simulink model "Lightning_McSeas_Dashboard"  (R2021b)
settings: Solver=VariableStepAuto  StartTime=0.0  StopTime=inf  RelTol=1e-3
undefined symbols (not defined in the file): canChannel
libraries: canlib x10, canmsglib x10
(part 2 of 2)

== system Lightning_McSeas_Dashboard/Battery Definiton ==
  note: Need to add the information for all of the voltages and temperatures maybe
  note: Battery definiton
  CAN Receive : canlib/CAN Receive  BlockHandle=5.0002  Device=MathWorks Virtual 1 (Channel 1)  DeviceMenu=MathWorks Virtual 1 (Channel 1)  ObjConstructor=canChannel('MathWorks', 'Virtual 1', 1)  EnableStandardIDsFilter=off  StdIDsCombo=Allow all  StandardIDs=1536  EnableExtendedIDsFilter=off  ExtIDsCombo=Allow all  ExtendedIDs=0  SampleTime=0.1  MsgsPerTimestep=all  InternalFilterUpdateStatus=on  BusOutput=off
      settings: SourceProductBaseCode=VN
  Dead : Terminator
  GPS Function : Subsystem  TreatAsAtomicUnit=on
  wires:
  CAN Receive/2 -> GPS Function/1(CAN Msg)
  GPS Function/1(Speed) -> Dead/1
  CAN Receive/1 -> GPS Function/Trigger

== system Lightning_McSeas_Dashboard/GPS Definintion ==
  note: GPS definiton
  CAN Receive : canlib/CAN Receive  BlockHandle=72.0009  Device=MathWorks Virtual 1 (Channel 1)  DeviceMenu=MathWorks Virtual 1 (Channel 1)  ObjConstructor=canChannel('MathWorks', 'Virtual 1', 1)  EnableStandardIDsFilter=off  StdIDsCombo=Allow all  StandardIDs=1536  EnableExtendedIDsFilter=off  ExtIDsCombo=Allow all  ExtendedIDs=0  SampleTime=0.1  MsgsPerTimestep=all  InternalFilterUpdateStatus=on  BusOutput=off
      settings: SourceProductBaseCode=VN
  GPS Function : Subsystem  TreatAsAtomicUnit=on
  Speed : Terminator
  wires:
  CAN Receive/2 -> GPS Function/1(CAN Msg)
  GPS Function/1(Speed) -> Speed/1
  CAN Receive/1 -> GPS Function/Trigger

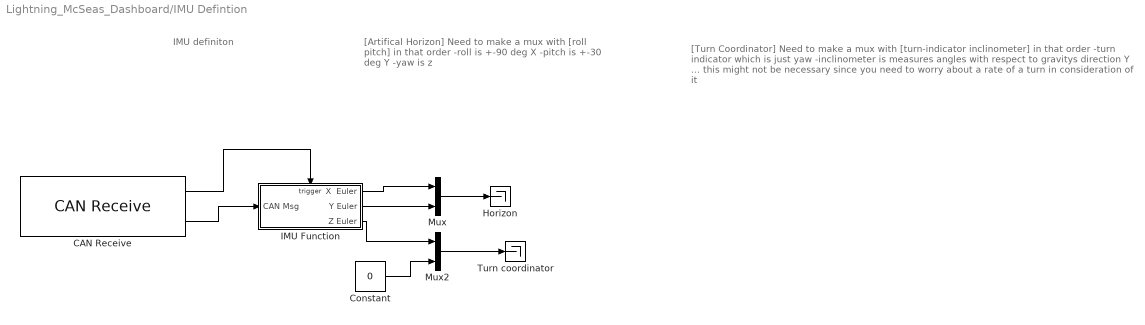
== system Lightning_McSeas_Dashboard/IMU Defintion ==
  note: [Turn Coordinator]
      | Need to make a mux with [turn-indicator inclinometer] in that order
      | -turn indicator which is just yaw
      |
      | -inclinometer is measures angles with respect to gravitys direction Y
      |
      | ... this might not be necessary since you need to worry about a rate of a turn in consideration of it
  note: [Artifical Horizon]
      | Need to make a mux with [roll pitch] in that order
      | -roll is +-90 deg X
      | -pitch is +-30 deg Y
      |
      | -yaw is z
  note: IMU definiton
  CAN Receive : canlib/CAN Receive  BlockHandle=38.0002  Device=MathWorks Virtual 1 (Channel 1)  DeviceMenu=MathWorks Virtual 1 (Channel 1)  ObjConstructor=canChannel('MathWorks', 'Virtual 1', 1)  EnableStandardIDsFilter=off  StdIDsCombo=Allow all  StandardIDs=1536  EnableExtendedIDsFilter=off  ExtIDsCombo=Allow all  ExtendedIDs=0  SampleTime=0.1  MsgsPerTimestep=all  InternalFilterUpdateStatus=on  BusOutput=off
      settings: SourceProductBaseCode=VN
  Constant : Constant  Value=0
  Horizon : Terminator
  IMU Function : Subsystem  TreatAsAtomicUnit=on
  Mux : Mux  Inputs=2
  Mux2 : Mux  Inputs=2
  Turn coordinator : Terminator
  wires:
  CAN Receive/2 -> IMU Function/1(CAN Msg)
  IMU Function/2(Y Euler) -> Mux/2
  IMU Function/3(Z Euler) -> Mux2/1
  CAN Receive/1 -> IMU Function/Trigger
  IMU Function/1(X  Euler) -> Mux/1
  Mux/1 -> Horizon/1
  Mux2/1 -> Turn coordinator/1
  Constant/1 -> Mux2/2

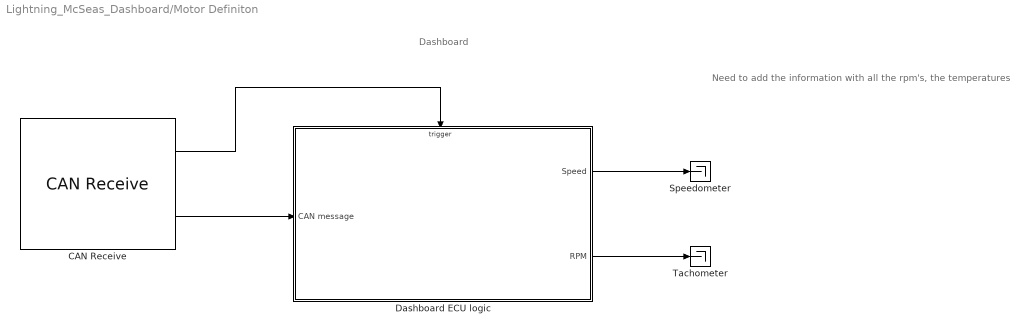
== system Lightning_McSeas_Dashboard/Motor Definiton ==
  note: Need to add the information with all the rpm's, the temperatures
  note: Dashboard
  CAN Receive : canlib/CAN Receive  BlockHandle=74.0002  Device=MathWorks Virtual 1 (Channel 2)  DeviceMenu=MathWorks Virtual 1 (Channel 2)  ObjConstructor=canChannel('MathWorks', 'Virtual 1', 2)  EnableStandardIDsFilter=off  StdIDsCombo=Block all  StandardIDs=0  EnableExtendedIDsFilter=off  ExtIDsCombo=Allow all  ExtendedIDs=[50 100]  SampleTime=0.01  MsgsPerTimestep=all  InternalFilterUpdateStatus=on  BusOutput=on
      settings: SourceProductBaseCode=VN
  Dashboard ECU logic : Subsystem  TreatAsAtomicUnit=on
  Speedometer : Terminator
  Tachometer : Terminator
  wires:
  CAN Receive/1 -> Dashboard ECU logic/Trigger
  CAN Receive/2 -> Dashboard ECU logic/1(CAN message)
  Dashboard ECU logic/2(RPM) -> Tachometer/1
  Dashboard ECU logic/1(Speed) -> Speedometer/1

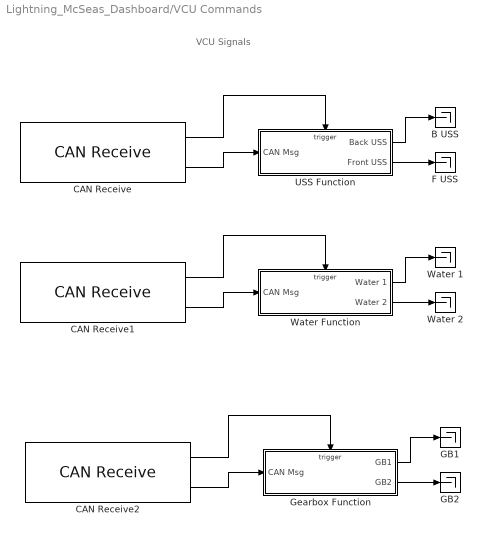
== system Lightning_McSeas_Dashboard/VCU Commands ==
  note: VCU Signals
  B USS : Terminator
  CAN Receive : canlib/CAN Receive  BlockHandle=72.0009  Device=MathWorks Virtual 1 (Channel 1)  DeviceMenu=MathWorks Virtual 1 (Channel 1)  ObjConstructor=canChannel('MathWorks', 'Virtual 1', 1)  EnableStandardIDsFilter=off  StdIDsCombo=Allow all  StandardIDs=1536  EnableExtendedIDsFilter=off  ExtIDsCombo=Allow all  ExtendedIDs=0  SampleTime=0.1  MsgsPerTimestep=all  InternalFilterUpdateStatus=on  BusOutput=off
      settings: SourceProductBaseCode=VN
  CAN Receive1 : canlib/CAN Receive  BlockHandle=72.0009  Device=MathWorks Virtual 1 (Channel 1)  DeviceMenu=MathWorks Virtual 1 (Channel 1)  ObjConstructor=canChannel('MathWorks', 'Virtual 1', 1)  EnableStandardIDsFilter=off  StdIDsCombo=Allow all  StandardIDs=1536  EnableExtendedIDsFilter=off  ExtIDsCombo=Allow all  ExtendedIDs=0  SampleTime=0.1  MsgsPerTimestep=all  InternalFilterUpdateStatus=on  BusOutput=off
      settings: SourceProductBaseCode=VN
  CAN Receive2 : canlib/CAN Receive  BlockHandle=72.0009  Device=MathWorks Virtual 1 (Channel 1)  DeviceMenu=MathWorks Virtual 1 (Channel 1)  ObjConstructor=canChannel('MathWorks', 'Virtual 1', 1)  EnableStandardIDsFilter=off  StdIDsCombo=Allow all  StandardIDs=1536  EnableExtendedIDsFilter=off  ExtIDsCombo=Allow all  ExtendedIDs=0  SampleTime=0.1  MsgsPerTimestep=all  InternalFilterUpdateStatus=on  BusOutput=off
      settings: SourceProductBaseCode=VN
  F USS : Terminator
  GB1 : Terminator
  GB2 : Terminator
  Gearbox Function : Subsystem  TreatAsAtomicUnit=on
  USS Function : Subsystem  TreatAsAtomicUnit=on
  Water 1 : Terminator
  Water 2 : Terminator
  Water Function : Subsystem  TreatAsAtomicUnit=on
  wires:
  CAN Receive/2 -> USS Function/1(CAN Msg)
  CAN Receive/1 -> USS Function/Trigger
  USS Function/1(Back USS) -> B USS/1
  USS Function/2(Front USS) -> F USS/1
  Water Function/1(Water 1) -> Water 1/1
  Water Function/2(Water 2) -> Water 2/1
  CAN Receive1/2 -> Water Function/1(CAN Msg)
  CAN Receive1/1 -> Water Function/Trigger
  CAN Receive2/1 -> Gearbox Function/Trigger
  Gearbox Function/1(GB1) -> GB1/1
  Gearbox Function/2(GB2) -> GB2/1
  CAN Receive2/2 -> Gearbox Function/1(CAN Msg)

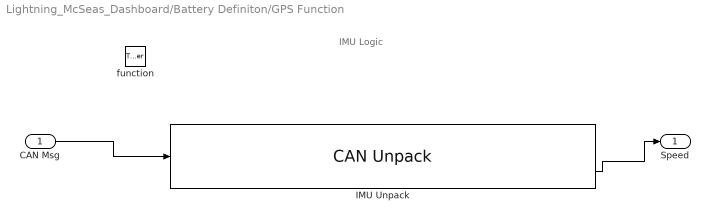
== system Lightning_McSeas_Dashboard/Battery Definiton/GPS Function ==
  note: IMU Logic
  CAN Msg : Inport
  function : TriggerPort  TriggerType=function-call  VariantControl=(inherit)
  IMU Unpack : canmsglib/CAN Unpack  CANdbFile=C:\Users\jerod\OneDrive\Documents\School-Files\Boat_Team\GitHubFiles\PCAN-GPS_Symbols.dbc  MsgList=GPS_CourseSpeed  MsgName=GPS_CourseSpeed  MsgIDType=Standard (11-bit identifier)  MsgIdentifier=1569  MsgLength=8  SignalInfo={'GPS_Course','0','32','LE','single','Standard','0','1','0','-3.4e+38','3.4e+38';'GPS_Speed','32','32','LE','single','Standard','0','1','0','-3.4e+38','3.4e+38'}  IDPort=off  TimestampPort=off  ErrorPort=off  RemotePort=off  LengthPort=off  StatusPort=off  ApplyMinMax=off
      settings: SourceProductBaseCode=ME,XP,VN  DataFormat=CANdb specified signals
  Speed : Outport
  wires:
  IMU Unpack/2 -> Speed/1
  CAN Msg/1 -> IMU Unpack/1

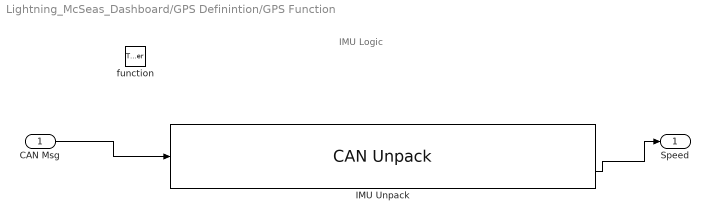
== system Lightning_McSeas_Dashboard/GPS Definintion/GPS Function ==
  note: IMU Logic
  CAN Msg : Inport
  function : TriggerPort  TriggerType=function-call  VariantControl=(inherit)
  IMU Unpack : canmsglib/CAN Unpack  CANdbFile=C:\Users\jerod\OneDrive\Documents\School-Files\Boat_Team\GitHubFiles\PCAN-GPS_Symbols.dbc  MsgList=GPS_CourseSpeed  MsgName=GPS_CourseSpeed  MsgIDType=Standard (11-bit identifier)  MsgIdentifier=1569  MsgLength=8  SignalInfo={ 'GPS_Course', '0', '32', 'LE', 'single', 'Standard', '0', '1', '0', '-3.4e+38', '3.4e+38'; 'GPS_Speed', '32', '32', 'LE', 'single', 'Standard', '0', '1', '0', '-3.4e+38', '3.4e+38' }  IDPort=off  TimestampPort=off  ErrorPort=off  RemotePort=off  LengthPort=off  StatusPort=off  ApplyMinMax=off
      settings: SourceProductBaseCode=ME,XP,VN  DataFormat=CANdb specified signals
  Speed : Outport
  wires:
  IMU Unpack/2 -> Speed/1
  CAN Msg/1 -> IMU Unpack/1

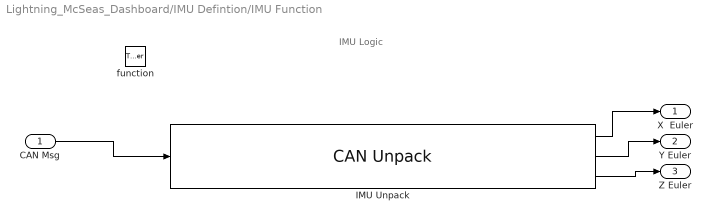
== system Lightning_McSeas_Dashboard/IMU Defintion/IMU Function ==
  note: IMU Logic
  CAN Msg : Inport
  function : TriggerPort  TriggerType=function-call  VariantControl=(inherit)
  IMU Unpack : canmsglib/CAN Unpack  CANdbFile=C:\Users\jerod\OneDrive\Documents\School-Files\Boat_Team\GitHubFiles\LPMS_IMU.dbc  MsgList=IMU_Euler_Angles  MsgName=IMU_Euler_Angles  MsgIDType=Standard (11-bit identifier)  MsgIdentifier=1301  MsgLength=8  SignalInfo={'Euler_X','0','16','LE','unsigned','Standard','0','0.01','0','-180','180';'Euler_Y','16','16','LE','unsigned','Standard','0','0.01','0','-90','90';'Euler_Z','32','16','LE','unsigned','Standard','0','0.01','0','-180','180'}  IDPort=off  TimestampPort=off  ErrorPort=off  RemotePort=off  LengthPort=off  StatusPort=off  ApplyMinMax=off
      settings: SourceProductBaseCode=ME,XP,VN  DataFormat=CANdb specified signals
  X  Euler : Outport
  Y Euler : Outport  Port=2
  Z Euler : Outport  Port=3
  wires:
  IMU Unpack/3 -> Z Euler/1
  IMU Unpack/1 -> X  Euler/1
  IMU Unpack/2 -> Y Euler/1
  CAN Msg/1 -> IMU Unpack/1

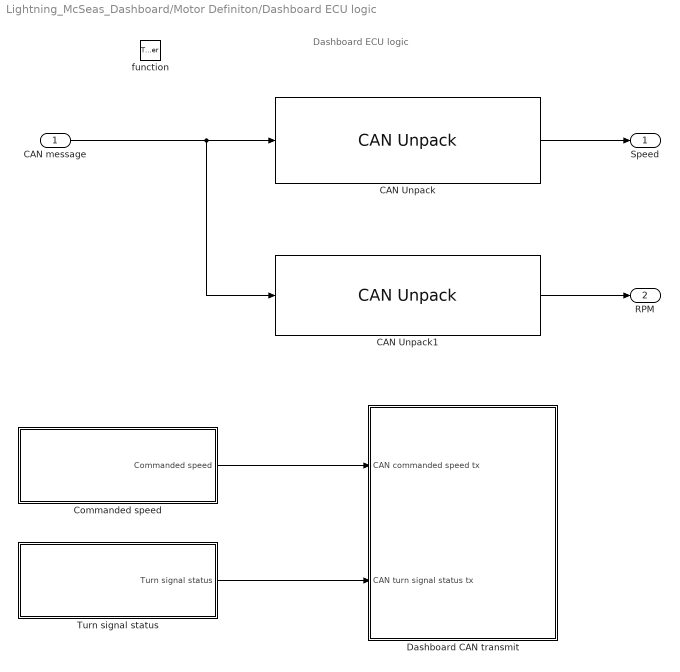
== system Lightning_McSeas_Dashboard/Motor Definiton/Dashboard ECU logic ==
  note: Dashboard ECU logic
  CAN message : Inport
  function : TriggerPort  TriggerType=function-call  VariantControl=Variant
  CAN Unpack : canmsglib/CAN Unpack  CANdbFile=H:\VNT_Project\Cruise_Control\candatabase\canConnectivityForVehicle.dbc  MsgList=SpeedMessage  MsgName=SpeedMessage  MsgIDType=Extended (29-bit identifier)  MsgIdentifier=256  MsgLength=8  SignalInfo={'Speed','0','64','LE','double','Standard','0','1','0','0','100'}  IDPort=off  TimestampPort=off  ErrorPort=off  RemotePort=off  LengthPort=off  StatusPort=off  ApplyMinMax=off
      settings: SourceProductBaseCode=ME,XP,VN  DataFormat=CANdb specified signals
  CAN Unpack1 : canmsglib/CAN Unpack  CANdbFile=H:\VNT_Project\Cruise_Control\candatabase\canConnectivityForVehicle.dbc  MsgList=RPMMessage  MsgName=RPMMessage  MsgIDType=Extended (29-bit identifier)  MsgIdentifier=2048  MsgLength=8  SignalInfo={'RPM','0','64','LE','double','Standard','0','1','0','0','10000'}  IDPort=off  TimestampPort=off  ErrorPort=off  RemotePort=off  LengthPort=off  StatusPort=off  ApplyMinMax=off
      settings: SourceProductBaseCode=ME,XP,VN  DataFormat=CANdb specified signals
  Commanded speed : Subsystem
  Dashboard CAN transmit : Subsystem
  Turn signal status : Subsystem
  Speed : Outport  VectorParamsAs1DForOutWhenUnconnected=off
  RPM : Outport  Port=2  VectorParamsAs1DForOutWhenUnconnected=off
  wires:
  CAN message/1 -> CAN Unpack1/1, CAN Unpack/1
  Turn signal status/1(Turn signal status) -> Dashboard CAN transmit/2(CAN turn signal status tx)
  Commanded speed/1(Commanded speed) -> Dashboard CAN transmit/1(CAN commanded speed tx)
  CAN Unpack/1 -> Speed/1
  CAN Unpack1/1 -> RPM/1

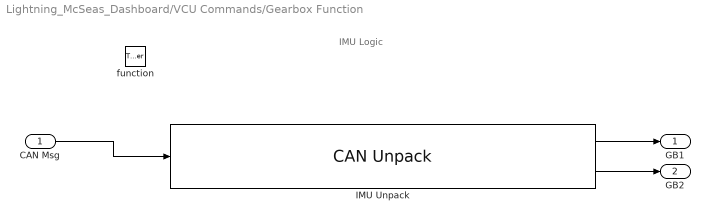
== system Lightning_McSeas_Dashboard/VCU Commands/Gearbox Function ==
  note: IMU Logic
  CAN Msg : Inport
  function : TriggerPort  TriggerType=function-call  VariantControl=(inherit)
  IMU Unpack : canmsglib/CAN Unpack  CANdbFile=C:\Users\jerod\OneDrive\Documents\School-Files\Boat_Team\GitHubFiles\LPMS_IMU.dbc  MsgList=Gearbox_Temps  MsgName=Gearbox_Temps  MsgIDType=Standard (11-bit identifier)  MsgIdentifier=3  MsgLength=8  SignalInfo={ 'Gearbox1', '0', '16', 'LE', 'unsigned', 'Standard', '0', '1', '0', '-Inf', 'Inf'; 'Gearbox2', '16', '16', 'LE', 'unsigned', 'Standard', '0', '1', '0', '-Inf', 'Inf' }  IDPort=off  TimestampPort=off  ErrorPort=off  RemotePort=off  LengthPort=off  StatusPort=off  ApplyMinMax=off
      settings: SourceProductBaseCode=ME,XP,VN  DataFormat=CANdb specified signals
  GB1 : Outport
  GB2 : Outport  Port=2
  wires:
  IMU Unpack/1 -> GB1/1
  IMU Unpack/2 -> GB2/1
  CAN Msg/1 -> IMU Unpack/1

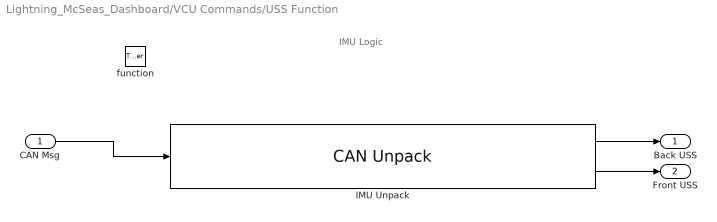
== system Lightning_McSeas_Dashboard/VCU Commands/USS Function ==
  note: IMU Logic
  CAN Msg : Inport
  function : TriggerPort  TriggerType=function-call  VariantControl=(inherit)
  IMU Unpack : canmsglib/CAN Unpack  CANdbFile=C:\Users\jerod\OneDrive\Documents\School-Files\Boat_Team\LPMS_IMU.dbc  MsgList=UltraSonic_Voltage  MsgName=UltraSonic_Voltage  MsgIDType=Standard (11-bit identifier)  MsgIdentifier=1  MsgLength=8  SignalInfo={ 'BackSensorReading', '16', '1', 'LE', 'unsigned', 'Standard', '0', '1', '0', '-Inf', 'Inf'; 'FrontSensorReading', '0', '16', 'LE', 'unsigned', 'Standard', '0', '1', '0', '-Inf', 'Inf' }  IDPort=off  TimestampPort=off  ErrorPort=off  RemotePort=off  LengthPort=off  StatusPort=off  ApplyMinMax=off
      settings: SourceProductBaseCode=ME,XP,VN  DataFormat=CANdb specified signals
  Back USS : Outport
  Front USS : Outport  Port=2
  wires:
  IMU Unpack/1 -> Back USS/1
  IMU Unpack/2 -> Front USS/1
  CAN Msg/1 -> IMU Unpack/1

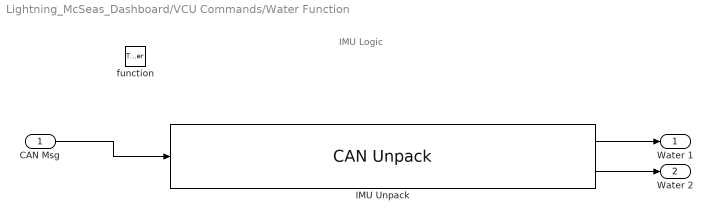
== system Lightning_McSeas_Dashboard/VCU Commands/Water Function ==
  note: IMU Logic
  CAN Msg : Inport
  function : TriggerPort  TriggerType=function-call  VariantControl=(inherit)
  IMU Unpack : canmsglib/CAN Unpack  CANdbFile=C:\Users\jerod\OneDrive\Documents\School-Files\Boat_Team\GitHubFiles\LPMS_IMU.dbc  MsgList=Water_Sensor_V_H  MsgName=Water_Sensor_V_H  MsgIDType=Standard (11-bit identifier)  MsgIdentifier=2  MsgLength=8  SignalInfo={ 'Water_Sensor_1', '0', '1', 'LE', 'unsigned', 'Standard', '0', '1', '0', '-Inf', 'Inf'; 'Water_Sensor_2', '1', '1', 'LE', 'unsigned', 'Standard', '0', '1', '0', '-Inf', 'Inf' }  IDPort=off  TimestampPort=off  ErrorPort=off  RemotePort=off  LengthPort=off  StatusPort=off  ApplyMinMax=off
      settings: SourceProductBaseCode=ME,XP,VN  DataFormat=CANdb specified signals
  Water 1 : Outport
  Water 2 : Outport  Port=2
  wires:
  IMU Unpack/1 -> Water 1/1
  IMU Unpack/2 -> Water 2/1
  CAN Msg/1 -> IMU Unpack/1

== system Lightning_McSeas_Dashboard/Motor Definiton/Dashboard ECU logic/Commanded speed ==
  note: Commanded speed
  Speed command : Constant  Value=61.59375  OutDataTypeStr=double  SampleTime=Inf
  Zero-Order Hold : ZeroOrderHold  SampleTime=-1
  Commanded speed : Outport  VectorParamsAs1DForOutWhenUnconnected=off
  wires:
  Speed command/1 -> Zero-Order Hold/1
  Zero-Order Hold/1 -> Commanded speed/1

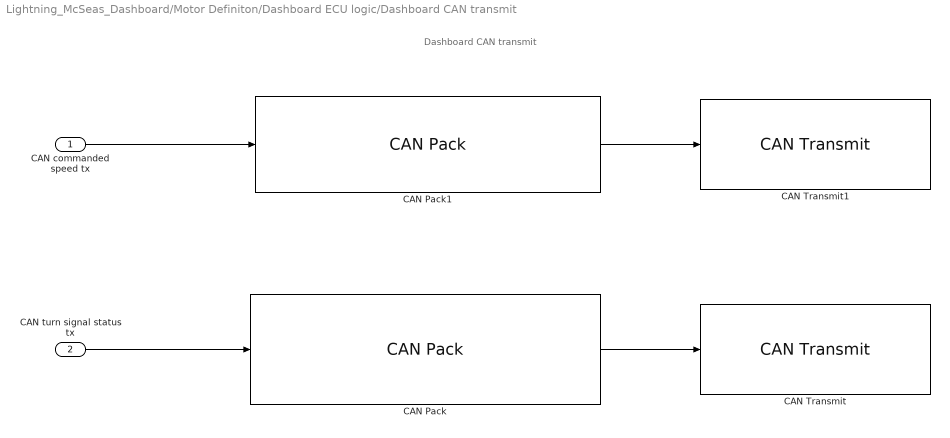
== system Lightning_McSeas_Dashboard/Motor Definiton/Dashboard ECU logic/Dashboard CAN transmit ==
  note: Dashboard CAN transmit
  CAN commanded speed tx : Inport
  CAN turn signal status tx : Inport  Port=2
  CAN Pack : canmsglib/CAN Pack  CANdbFile=H:\VNT_Project\Cruise_Control\candatabase\canConnectivityForVehicle.dbc  MsgList=TurnSignalStatusMessage  MsgName=TurnSignalStatusMessage  MsgIDType=Extended (29-bit identifier)  MsgIdentifier=1536  MsgLength=1  Remote=off  ApplyMinMax=off  BusOutput=on  SignalInfo={'TurnSignalStatus','0','3','LE','unsigned','Standard','0','1','0','1','3'}
      settings: SourceProductBaseCode=ME,XP,VN  DataFormat=CANdb specified signals
  CAN Pack1 : canmsglib/CAN Pack  CANdbFile=H:\VNT_Project\Cruise_Control\candatabase\canConnectivityForVehicle.dbc  MsgList=SpeedCommandMessage  MsgName=SpeedCommandMessage  MsgIDType=Extended (29-bit identifier)  MsgIdentifier=1024  MsgLength=8  Remote=off  ApplyMinMax=off  BusOutput=on  SignalInfo={'SpeedCommand','0','64','LE','double','Standard','0','1','0','0','100'}
      settings: SourceProductBaseCode=ME,XP,VN  DataFormat=CANdb specified signals
  CAN Transmit : canlib/CAN Transmit  BlockHandle=40.0009  Device=MathWorks Virtual 1 (Channel 1)  DeviceMenu=MathWorks Virtual 1 (Channel 1)  ObjConstructor=canChannel('MathWorks', 'Virtual 1', 1)  EnableEventTransmit=off  EnablePeriodicTransmit=on  MessagePeriod=0.01
      settings: SourceProductBaseCode=VN
  CAN Transmit1 : canlib/CAN Transmit  BlockHandle=41.0009  Device=MathWorks Virtual 1 (Channel 1)  DeviceMenu=MathWorks Virtual 1 (Channel 1)  ObjConstructor=canChannel('MathWorks', 'Virtual 1', 1)  EnableEventTransmit=off  EnablePeriodicTransmit=on  MessagePeriod=0.01
      settings: SourceProductBaseCode=VN
  wires:
  CAN commanded speed tx/1 -> CAN Pack1/1
  CAN Pack/1 -> CAN Transmit/1
  CAN turn signal status tx/1 -> CAN Pack/1
  CAN Pack1/1 -> CAN Transmit1/1

== system Lightning_McSeas_Dashboard/Motor Definiton/Dashboard ECU logic/Turn signal status ==
  note: Turn signal status
  Turn signal : Constant  Value=2  OutDataTypeStr=double
  Zero-Order Hold : ZeroOrderHold  SampleTime=-1
  Turn signal status : Outport  VectorParamsAs1DForOutWhenUnconnected=off
  wires:
  Turn signal/1 -> Zero-Order Hold/1
  Zero-Order Hold/1 -> Turn signal status/1
